simulink model "sl_subsys_fcncall6"  (Simulink 7.6)
settings: Solver=FixedStepDiscrete  StartTime=0.0  StopTime=10.0  FixedStep=1  RelTol=1e-3
Description:
  | Multiple initiators of a function-call subsystem
  | 
  | The following function-call subsystem is called by two different function-call
  | initiators (Chart1 and Chart2). The data connection between Chart1/out1 and
  | Chart2/d1 guarantees that Chart1 executes before Chart2.
  | 
  | Caution needs to be taken when creating function-call subsystems with
  | multiple callers. For example, if you remove the data connection between Chart1 and
  | Chart2, then you need to add priorities to Chart1 and Chart2 using the block
  | property dialogs to specify the relative execution order of these blocks. Failure
  | to do so will mean that your model's execution, in general, will be
  | ambiguous. However, Simulink does not error out for this condition because
  | it may be valid for specific cases. As an example, if all states are removed from
  | f() and the line from Chart1/out1 to Chart2/d1 is deleted, then the order in which
  | Chart1 and Chart2 execute does not matter.
settings Model: Creator=The MathWorks Inc.  CovMetricSettings=d  ExtModeAutoUpdateStatusClock=off
settings OptimizationCC: BlockReduction=off  BooleanDataType=off  InlineInvariantSignals=on  InitFltsAndDblsToZero=on
settings DebuggingCC: SaveWithParameterizedLinksMsg=none  SignalResolutionControl=TryResolveAllWithWarning  SolverPrmCheckMsg=none  MultiTaskDSMMsg=warning  MultiTaskCondExecSysMsg=none
settings HardwareCC: TargetUnknown=on
settings SFSimCC: SimParseCustomCode=off
settings RTWCC: IncludeERTFirstTime=on
settings CodeAppCC: CustomSymbolStrFcn=$F$N$M
settings GRTTargetCC: TargetFcnLib=ansi_tfl_tmw.mat

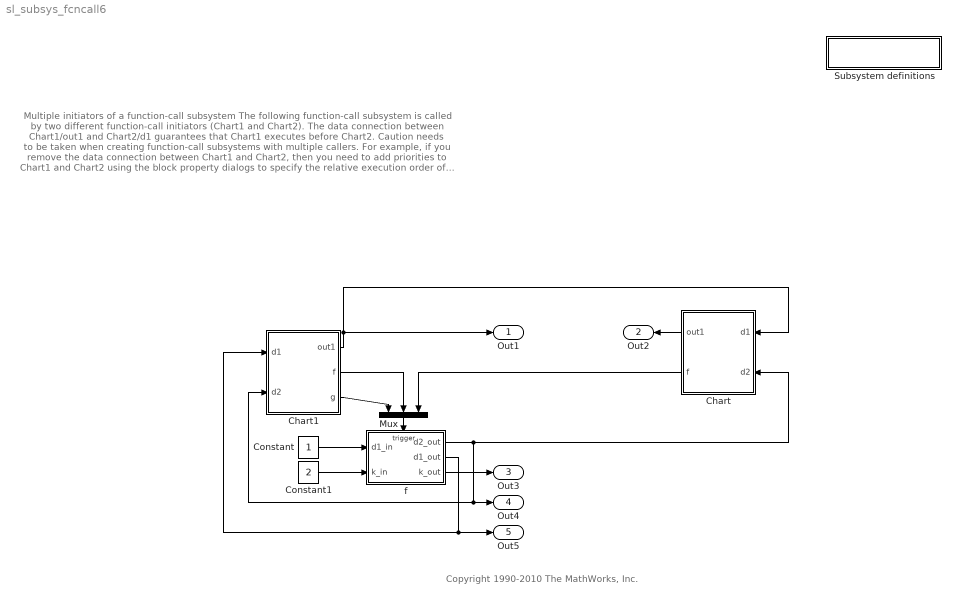
== system sl_subsys_fcncall6 ==
  note: Multiple initiators of a function-call subsystem
      |
      | The following function-call subsystem is called by two different function-call
      | initiators (Chart1 and Chart2). The data connection between Chart1/out1 and
      | Chart2/d1 guarantees that Chart1 executes before Chart2.
      |
      | Caution needs to be taken when creating function-call subsystems with
      | multiple callers. For example, if you remove the data connection between Chart1 and
      | Chart2, then you need to add priorities to Chart1 and Chart2 using the block
      | property dialogs to specify the relative execution order of these blocks. Failure
      | to do so will mean that your model's execution, in general, will be
      | ambiguous. However, Simulink does not error out for this condition because
      | it may be valid for specific cases. As an example, if all states are removed from
      | f() and the line from Chart1/out1 to Chart2/d1 is deleted, then the order in which
      | Chart1 and Chart2 execute does not matter.
  note: Copyright 1990-2010 The MathWorks, Inc.
  " Subsystem definitions" : Subsystem
      settings: OpenFcn=helpview([matlabroot,'/toolbox/simulink/simdemos/simfeatures/html/sl_subsys_definitions.html']);
      mask Display: disp('Subsystem\ndefinitions')
  Chart : Stateflow chart  TreatAsAtomicUnit=on
  Chart1 : Stateflow chart  TreatAsAtomicUnit=on
  Constant : Constant
  Constant1 : Constant  Value=2
  Mux : Mux  Inputs=3
  f : Subsystem  TreatAsAtomicUnit=on
  Out1 : Outport
  Out2 : Outport  Port=2
  Out3 : Outport  Port=3
  Out4 : Outport  Port=4
  Out5 : Outport  Port=5
  wires:
  f/1(d2_out) -> Out4/1, Chart1/2(d2), Chart/2(d2)
  Chart1/1(out1) -> Out1/1, Chart/1(d1)
  Mux/1 -> f/Trigger
  Chart1/3(g) -> Mux/1
  Chart1/2(f) -> Mux/2
  Chart/1(out1) -> Out2/1
  Chart/2(f) -> Mux/3
  f/2(d1_out) -> Out5/1, Chart1/1(d1)
  f/3(k_out) -> Out3/1
  Constant/1 -> f/1(d1_in)
  Constant1/1 -> f/2(k_in)

== system sl_subsys_fcncall6/ Subsystem definitions ==

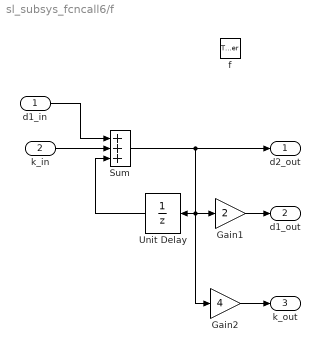
== system sl_subsys_fcncall6/f ==
  d1_in : Inport
  k_in : Inport  Port=2
  f : TriggerPort  TriggerType=function-call
  Gain1 : Gain  Gain=2  SaturateOnIntegerOverflow=on  OutDataTypeStr=Inherit: Same as input  ParamDataTypeStr=Inherit: Same as input
  Gain2 : Gain  Gain=4  SaturateOnIntegerOverflow=on  OutDataTypeStr=Inherit: Same as input  ParamDataTypeStr=Inherit: Same as input
  Sum : Sum  Inputs=+++  SaturateOnIntegerOverflow=on  InputSameDT=on  OutDataTypeStr=Inherit: Same as first input
  Unit Delay : UnitDelay  SampleTime=-1
  d2_out : Outport
  d1_out : Outport  Port=2
  k_out : Outport  Port=3
  wires:
  Unit Delay/1 -> Sum/3
  Sum/1 -> Unit Delay/1, Gain1/1, Gain2/1, d2_out/1
  d1_in/1 -> Sum/1
  Gain1/1 -> d1_out/1
  Gain2/1 -> k_out/1
  k_in/1 -> Sum/2

== stateflow chart Chart1 ==
  state one/
    entry: f; out1= d1+d2;
  state two/
    entry: g; out1=d1-d2;
  one -> two
  two -> one
  (default) -> one
  data: d1 input double; d2 input double; out1 output double
  events: f output FUNCTION_CALL_EVENT; g output FUNCTION_CALL_EVENT

== stateflow chart Chart ==
  state one/
    entry:f;out1=d1+d2;
  state two/
    entry: f;out1=d1-d2;
  one -> two
  two -> one
  (default) -> one
  data: d1 input double; d2 input double; out1 output double; out local double
  events: f output FUNCTION_CALL_EVENT
